simulink model "Centrum_doswiadczalne_LS_posrednia"  (R2016a)
settings: Solver=FixedStepAuto  StartTime=0.0  StopTime=30  FixedStep=0.01  RelTol=1e-3
settings Model: Creator=agnpi  LastModifiedBy=agnpi

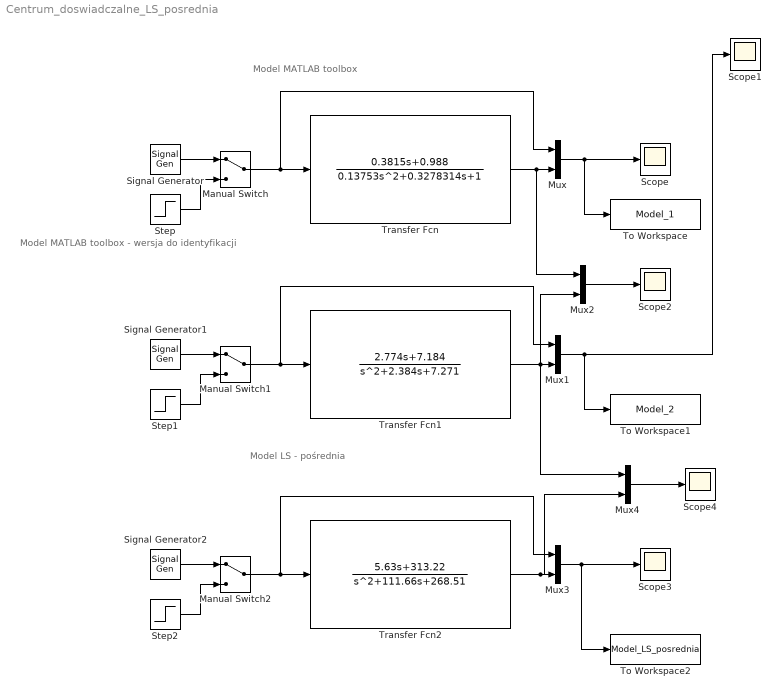
== system Centrum_doswiadczalne_LS_posrednia ==
  note: Model MATLAB toolbox - wersja do identyfikacji
  note: Model MATLAB toolbox
  note: Model LS - pośrednia
  Manual Switch : ManualSwitch
  Manual Switch1 : ManualSwitch
  Manual Switch2 : ManualSwitch
  Mux{,1..4} (5 alike) : Mux  Inputs=2
  Scope{,1..4} (5 alike) : Scope
  Signal Generator : SignalGenerator  WaveForm=square  Frequency=0.1
  Signal Generator1 : SignalGenerator  WaveForm=square  Frequency=0.1
  Signal Generator2 : SignalGenerator  WaveForm=square  Frequency=0.1
  Step : Step  Time=0  Before=-1  SampleTime=0
  Step1 : Step  Time=0  Before=-1  SampleTime=0
  Step2 : Step  Time=0  Before=-1  SampleTime=0
  To Workspace : ToWorkspace  VariableName=Model_1  SampleTime=-1
  To Workspace1 : ToWorkspace  VariableName=Model_2  SampleTime=-1
  To Workspace2 : ToWorkspace  VariableName=Model_LS_posrednia  SampleTime=-1
  Transfer Fcn : TransferFcn  Numerator=[0.3815 0.988]  Denominator=[0.13753 0.3278314 1]
  Transfer Fcn1 : TransferFcn  Numerator=[2.774 7.184]  Denominator=[1 2.384 7.271]
  Transfer Fcn2 : TransferFcn  Numerator=[0 5.63 313.22]  Denominator="[1 111.66  268.51]"
  wires:
  Transfer Fcn/1 -> Mux2/1, Mux/2
  Signal Generator/1 -> Manual Switch/1
  Mux/1 -> To Workspace/1, Scope/1
  Manual Switch/1 -> Mux/1, Transfer Fcn/1
  Step/1 -> Manual Switch/2
  Step1/1 -> Manual Switch1/2
  Manual Switch1/1 -> Mux1/1, Transfer Fcn1/1
  Signal Generator1/1 -> Manual Switch1/1
  Mux1/1 -> To Workspace1/1, Scope1/1
  Mux2/1 -> Scope2/1
  Signal Generator2/1 -> Manual Switch2/1
  Mux3/1 -> To Workspace2/1, Scope3/1
  Manual Switch2/1 -> Mux3/1, Transfer Fcn2/1
  Step2/1 -> Manual Switch2/2
  Transfer Fcn2/1 -> Mux4/2, Mux3/2
  Mux4/1 -> Scope4/1
  Transfer Fcn1/1 -> Mux4/1, Mux2/2, Mux1/2
